simulink model "LQR_simulation"  (R2019a)
settings: Solver=VariableStepAuto  StartTime=0.0  StopTime=24  RelTol=1e-3
values from neighbouring files (symbols this model uses):
  A = modeld.a    [LQR_initialization.m]    (also in LQ_observer_initialization.m; MPC_initialization.m = sysd.a; MagnetoShield_LQ_Initialization.m; MagnetoShield_PolePlacement_Initialization.m)
  B = modeld.b    [LQR_initialization.m]    (also in LQ_observer_initialization.m; MPC_initialization.m = sysd.b; MagnetoShield_LQ_Initialization.m; MagnetoShield_PolePlacement_Initialization.m)
  C = [1 0 0;0 0 1]    [LQR_initialization.m]    (also in LQ_observer_initialization.m = [1 0 0]; MPC_initialization.m = [1 0 0]; MagnetoShield_LQ_Initialization.m; MagnetoShield_PolePlacement_Initialization.m = [1 0 0])
  Ci = [1 0 0]    [LQR_initialization.m]    (also in MagnetoShield_LQ_Initialization.m)
  D = [0;0]    [LQR_initialization.m]    (also in LQ_observer_initialization.m = 0; MPC_initialization.m = 0; MagnetoShield_LQ_Initialization.m)
  i0 = 0.00301720799779    [MagnetoShield_Alternative_model.mat]    (also in MagnetoShield_Models_Greybox_SS model.mat = 0.0219057293333)
  K = dlqr(Ai,Bi,Qlq,Rlq)    [LQR_initialization.m]    (also in LQ_observer_initialization.m; MagnetoShield_LQ_Initialization.m; MagnetoShield_PolePlacement_Initialization.m = [0 0 0 1]*inv([Bi Ai*Bi Ai^2*Bi Ai^3*Bi])*phy)
  R = [0.001, 0.01]    [LQR_initialization.m]    (also in MagnetoShield_LQ_Initialization.m = diag([1.5815e-10,6.6217e-09]))
  Ts = 0.001    [LQR_initialization.m]    (also in LQ_observer_initialization.m = 0.002; MPC_initialization.m; MagnetoShield_LQ_Initialization.m = 0.0015; MagnetoShield_PolePlacement_Initialization.m = 0.0015)
  u0 = 0.633613679536    [MagnetoShield_Alternative_model.mat]    (also in MagnetoShield_Models_Greybox_SS model.mat = 4.62338933333)
  y0 = 0.012    [MagnetoShield_Alternative_model.mat]    (also in MagnetoShield_Models_Greybox_SS model.mat = 0.0143094466667)
undefined symbols (not defined in the file or in its folder): DiscIntNeverNeededParam, Discrete, Time
libraries: simulink x2, ctrlSharedLib x1
settings Model: Creator=jakub  LastModifiedBy=jakub

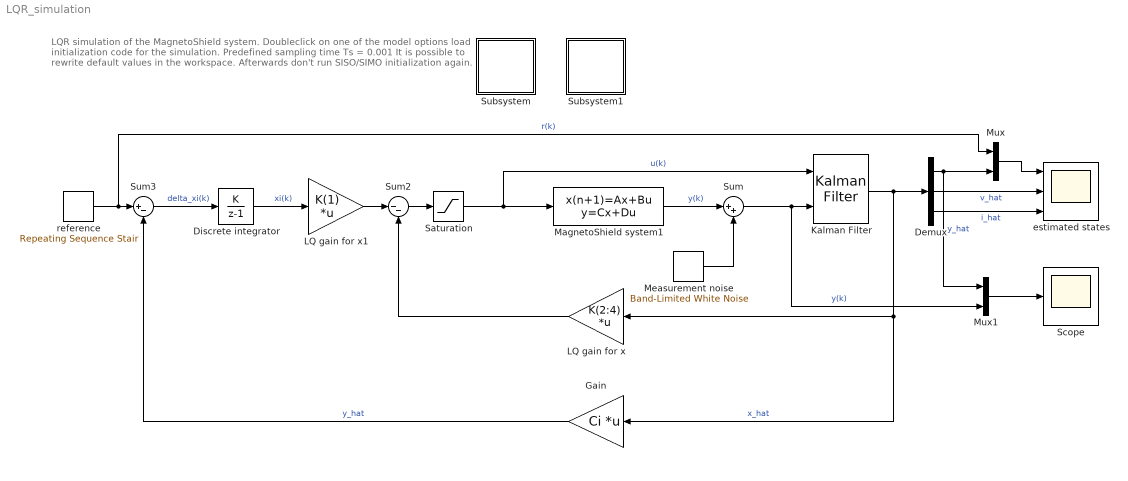
== system LQR_simulation ==
  note: LQR simulation of the  MagnetoShield system.
      | Doubleclick on one of the model options load initialization code for the simulation.
      | Predefined sampling time Ts = 0.001
      | It is possible to rewrite default values in the workspace.  Afterwards don't run SISO/SIMO
      | initialization again.
  Demux : Demux  Outputs=3
  Discrete integrator : DiscreteIntegrator  IntegratorMethod=Accumulation: Forward Euler  SampleTime=Ts  LimitOutput=on  ICPrevOutput=DiscIntNeverNeededParam  ICPrevScaledInput=DiscIntNeverNeededParam
  Gain : Gain  Gain=Ci  Multiplication=Matrix(K*u)
  Kalman Filter : ctrlSharedLib/Kalman Filter  TimeDomain=Discrete-Time  UseCurrentEstimator=on  ModelSource=Individual A, B, C, D matrices  ModelSourceVariable=ss(0.95,1,1,0,1)  A=A  B=B  C=C  D=D  NumberOfStates=1  NumberOfInputs=1  NumberOfOutputs=1  InitialEstimateSource=Dialog  X0=[0.017-y0;0;0-i0]  P0=10  UseK=off  UseGH=off  NumberOfProcessNoiseInputs=1  G=1  TimeInvariantG=on  H=0  TimeInvariantH=on  Q=Q  TimeInvariantQ=on  R=R  TimeInvariantR=on  N=0  TimeInvariantN=on  AddInputPort=on  AddEnablePort=off  OutputEstimatedY=off  OutputP=off  Ts=-1
  LQ gain for x : Gain  Gain=K(2:4)  Multiplication=Matrix(K*u)
  LQ gain for x1 : Gain  Gain=K(1)  Multiplication=Matrix(K*u)
  MagnetoShield system1 : DiscreteStateSpace  A=A  B=B  C=C  D=D  InitialCondition=[0.017-y0;0;0-i0]  SampleTime=Ts
  Measurement noise : simulink/Sources/Band-Limited White Noise  Cov=[(2*10^(-7))^2]  Ts=2*Ts  seed=[23341]
  Mux : Mux  Inputs=2
  Mux1 : Mux  Inputs=2
  Saturation : Saturate  UpperLimit=12-u0  LowerLimit=0-u0
  Scope : Scope
  Subsystem : Subsystem
      settings: OpenFcn=|
      | clear;close all;clc;
      | load '../../../matlab/examples/MagnetoShield/MagnetoShield_Models_Greybox_SS';
      | %% MagnetoShield - LQR simulation and control initialization for Simulink
      | 
      | order = 'SISO';                 % SISO - position / SIMO - position & current
      | Ts = 0.001;                    % Sampling of the Simulink simulation
      | 
      | % Matrices extraction from model
      | modeld=c2d(model,Ts);           % Discretized linear state-space model
      | A = modeld.a;                   % Extract A
      | B = modeld.b;                   % Extract B
      | Ci = [1 0 0];                   % Position is measured for integrator 'xi' computation
      | D = 0;
      | 
      | % Discrete augmented model with integrator state - unstable, unobservable
      | Ai = [1 -Ci;
      |       zeros(3,1) A];
      | Bi = [0;B];
      | 
      | % %Simulations
      | Qlq=diag([70 100 20 40]);      % State penalty matrix
      | Rlq=0.1;                       % Input penalty matrix
      | K=dlqr(Ai,Bi,Qlq,Rlq);         % LQ gain for system states
      | 
      | % Measurement matrices of state-space and Kalman filter gains
      | if order == 'SISO'                  % Setup if just position is measured
      |     C = [1 0 0];
      |     D = 0;
      |     Q = diag([0.0001, 100, 100]);   % Penalty of the model for Kalman filter
      |     R = 0.001;                     % Penalty of measurement for Kalman filter
      | 
      | elseif order == 'SIMO'             % Setup if position and current are measured
      |     C = [1 0 0;0 0 1];
      |     D = [0;0];
      |     Q = diag([0.0001, 100, 80]);   % Penalty of the model for Kalman filter
      |     R = [0.001, 0.01];             % Penalty of measurement for Kalman filter
      | end
      mask Display: disp('SISO')
  Subsystem1 : Subsystem
      settings: OpenFcn=|
      | clear;close all;clc;
      | load '../../../matlab/examples/MagnetoShield/MagnetoShield_Models_Greybox_SS';
      | %% MagnetoShield - LQR simulation and control initialization for Simulink
      | 
      | order = 'SIMO';                 % SISO - position / SIMO - position & current
      | Ts = 0.001;                    % Sampling of the Simulink simulation
      | 
      | % Matrices extraction from model
      | modeld=c2d(model,Ts);           % Discretized linear state-space model
      | A = modeld.a;                   % Extract A
      | B = modeld.b;                   % Extract B
      | Ci = [1 0 0];                   % Position is measured for integrator 'xi' computation
      | D = 0;
      | 
      | % Discrete augmented model with integrator state - unstable, unobservable
      | Ai = [1 -Ci;
      |       zeros(3,1) A];
      | Bi = [0;B];
      | 
      | % LQ gain computation - the 1. tuning diverges in the simulations but is
      | % smoother in experiments:
      | %Simulations
      | Qlq=diag([70 100 20 40]);      % State penalty matrix
      | Rlq=0.1;                       % Input penalty matrix
      | K=dlqr(Ai,Bi,Qlq,Rlq);         % LQ gain for system states
      | 
      | % Measurement matrices of state-space and Kalman filter gains
      | if order == 'SISO'                  % Setup if just position is measured
      |     C = [1 0 0];
      |     D = 0;
      |     Q = diag([0.0001, 100, 100]);   % Penalty of the model for Kalman filter
      |     R = 0.001;                     % Penalty of measurement for Kalman filter
      | 
      | elseif order == 'SIMO'             % Setup if position and current are measured
      |     C = [1 0 0;0 0 1];
      |     D = [0;0];
      |     Q = diag([0.0001, 100, 80]);   % Penalty of the model for Kalman filter
      |     R = [0.001, 0.01];             % Penalty of measurement for Kalman filter
      | end
      mask Display: disp('SIMO')
  Sum : Sum  Inputs=|++
  Sum2 : Sum  Inputs=|--
  Sum3 : Sum  Inputs=|+-
  estimated states : Scope  NumInputPorts=3
  reference : simulink/Sources/Repeating Sequence Stair  OutValues=[ones(1,2000)*(0.013-y0) ones(1,2000)*(0.016-y0) ones(1,2000)*(0.012-y0)].'  tsamp=Ts  OutMin=[]  OutMax=[]  OutDataTypeStr=double  OutputDataTypeScalingMode=double  OutDataType=fixdt(0,8)  ConRadixGroup=Best Precision: Vector-wise  OutScaling=2^-12
  wires:
  LQ gain for x/1 -> Sum2/2
  LQ gain for x1/1 -> Sum2/1
  Sum3/1 -> Discrete integrator/1  "delta_xi(k)"
  reference/1 -> Mux/1, Sum3/1  "r(k)"
  Discrete integrator/1 -> LQ gain for x1/1  "xi(k)"
  Saturation/1 -> MagnetoShield system1/1, Kalman Filter/1  "u(k)"
  Kalman Filter/1 -> Gain/1, LQ gain for x/1, Demux/1  "x_hat"
  Sum2/1 -> Saturation/1
  Gain/1 -> Sum3/2  "y_hat"
  Sum/1 -> Mux1/2, Kalman Filter/2  "y(k)"
  Measurement noise/1 -> Sum/2
  Mux/1 -> estimated states/1
  Demux/1 -> Mux/2, Mux1/1  "y_hat"
  Demux/2 -> estimated states/2  "v_hat"
  Demux/3 -> estimated states/3  "i_hat"
  Mux1/1 -> Scope/1
  MagnetoShield system1/1 -> Sum/1  "y(k)"

== system LQR_simulation/Subsystem ==

== system LQR_simulation/Subsystem1 ==
